simulink model "test"  (R2020b)
settings: Solver=FixedStepAuto  StartTime=0.0  StopTime=2000  RelTol=1e-3  EnableMultiTasking=on
undefined symbols (not defined in the file or in its folder): DiscIntNeverNeededParam
libraries: bbblueCommlib x15, simulink x7, bbblueBasicLib x4, bbblueSensorLib x1
settings Model: SimulationMode=external  ExtModeArchiveFileName=asd  ExtModeArchiveDirName=C:\Users\Zein\Desktop\gui  ExtModeIncDirWhenArm=on  Creator=Zein  LastModifiedBy=Zein
settings SolverCC: PositivePriorityOrder=on
settings OptimizationCC: EnhancedBackFolding=on  PassReuseOutputArgsAs=Individual arguments  ZeroExternalMemoryAtStartup=off  ZeroInternalMemoryAtStartup=off  MaxStackSize=64  OptimizeBlockOrder=speed  DifferentSizesBufferReuse=on  OptimizationCustomize=off  EfficientTunableParamExpr=on
settings DebuggingCC: ParameterTunabilityLossMsg=error
settings HardwareCC: ProdBitPerPointer=32  ProdBitPerSizeT=32  ProdBitPerPtrDiffT=32  ProdLargestAtomicInteger=Long  ProdLargestAtomicFloat=Double  ProdWordSize=32  ProdHWDeviceType=ARM Compatible->ARM Cortex
settings SFSimCC: MATLABDynamicMemAlloc=off
settings RTWCC: Description=Embedded Coder  SystemTargetFile=ert.tlc  HardwareBoard=BeagleBone Blue  TLCOptions="-aInlineSetEventsForThisBaseRateFcn=TLC_FALSE -aSuppressMultiTaskScheduler=TLC_FALSE  -aRateBasedStepFcn=0"  TemplateMakefile=ert_default_tmf  Toolchain=GNU GCC BeagleBone Blue
settings CodeAppCC: ForceParamTrailComments=on  IgnoreCustomStorageClasses=off  OperatorAnnotations=on  SimulinkDataObjDesc=on  SFDataObjDesc=on  InsertBlockDesc=on
settings ERTTargetCC: MatFileLogging=on  SupportVariableSizeSignals=on

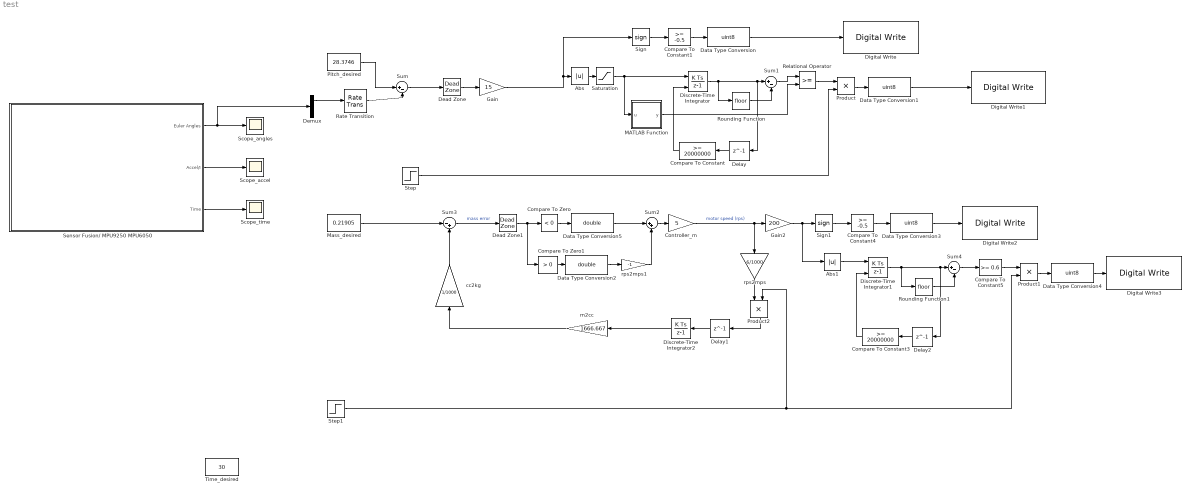
== system test ==
  Abs : Abs
  Abs1 : Abs
  Compare To Constant : simulink/Logic and Bit Operations/Compare To Constant  relop=>=  const=20000000  OutDataTypeStr=boolean
  Compare To Constant1 : simulink/Logic and Bit Operations/Compare To Constant  relop=>=  const=-0.5  OutDataTypeStr=boolean
  Compare To Constant3 : simulink/Logic and Bit Operations/Compare To Constant  relop=>=  const=20000000  OutDataTypeStr=boolean
  Compare To Constant4 : simulink/Logic and Bit Operations/Compare To Constant  relop=>=  const=-0.5  OutDataTypeStr=boolean
  Compare To Constant5 : simulink/Logic and Bit Operations/Compare To Constant  relop=>=  const=0.6  OutDataTypeStr=uint8
  Compare To Zero : simulink/Logic and Bit Operations/Compare To Zero  relop=<  OutDataTypeStr=boolean
  Compare To Zero1 : simulink/Logic and Bit Operations/Compare To Zero  relop=>  OutDataTypeStr=boolean
  Controller_m : Gain  Gain=5
  Data Type Conversion{,1,3..4} (4 alike) : DataTypeConversion  OutDataTypeStr=uint8
  Data Type Conversion2 : DataTypeConversion  OutDataTypeStr=double
  Data Type Conversion5 : DataTypeConversion  OutDataTypeStr=double
  Dead Zone : DeadZone  LowerValue=-5  UpperValue=5  SaturateOnIntegerOverflow=on
  Dead Zone1 : DeadZone  LowerValue=-0.0001  UpperValue=0.0001  SaturateOnIntegerOverflow=on
  Delay : Delay  DelayLength=1
  Delay1 : Delay  DelayLength=1  SampleTime=1/5000
  Delay2 : Delay  DelayLength=1
  Demux : Demux  Outputs=3
  Digital Write : bbblueBasicLib/Digital Write  GPIOSelect=GPIO3_1  Pin=49  Direction=output
      settings: SourceProductBaseCode=SC_BEAGLEBONE_BLUE
  Digital Write1 : bbblueBasicLib/Digital Write  GPIOSelect=GPIO3_2  Pin=49  Direction=output
      settings: SourceProductBaseCode=SC_BEAGLEBONE_BLUE
  Digital Write2 : bbblueBasicLib/Digital Write  GPIOSelect=GPIO1_17  Pin=49  Direction=output
      settings: SourceProductBaseCode=SC_BEAGLEBONE_BLUE
  Digital Write3 : bbblueBasicLib/Digital Write  GPIOSelect=GPIO1_25  Pin=49  Direction=output
      settings: SourceProductBaseCode=SC_BEAGLEBONE_BLUE
  Discrete-Time Integrator : DiscreteIntegrator  ExternalReset=rising  SampleTime=1/5000  ICPrevOutput=DiscIntNeverNeededParam  ICPrevScaledInput=DiscIntNeverNeededParam
  Discrete-Time Integrator1 : DiscreteIntegrator  ExternalReset=rising  SampleTime=1/5000  ICPrevOutput=DiscIntNeverNeededParam  ICPrevScaledInput=DiscIntNeverNeededParam
  Discrete-Time Integrator2 : DiscreteIntegrator  SampleTime=1/5000  ICPrevOutput=DiscIntNeverNeededParam  ICPrevScaledInput=DiscIntNeverNeededParam
  Gain : Gain  Gain=15
  Gain2 : Gain  Gain=200
  MATLAB Function : MATLAB Function  TreatAsAtomicUnit=on
  Mass_desired : Constant  Value=0.21905
  Pitch_desired : Constant  Value=28.3746
  Product : Product
  Product1 : Product
  Product2 : Product
  Rate Transition : RateTransition
  Relational Operator : RelationalOperator  OutDataTypeStr=boolean  RndMeth=Round
  Rounding Function : Rounding
  Rounding Function1 : Rounding
  Saturation : Saturate  UpperLimit=1000  LowerLimit=0
  Scope_accel : Scope
  Scope_angles : Scope
  Scope_time : Scope
  Sensor Fusion/ MPU9250 MPU6050 : Subsystem
  Sign : Signum
  Sign1 : Signum
  Step : Step  Time=31
  Step1 : Step  Time=3
  Sum : Sum  Inputs=|+-
  Sum1 : Sum  Inputs=|+-
  Sum2 : Sum  Inputs=|++
  Sum3 : Sum  Inputs=|-+
  Sum4 : Sum  Inputs=|+-
  Time_desired : Constant  Value=30
  cc2kg : Gain  Gain=1/1000
  m2cc : Gain  Gain=1666.667
  rps2mps : Gain  Gain=6/1000
  rps2mps1 : Gain  Gain=-1
  wires:
  Sensor Fusion/ MPU9250 MPU6050/1(Euler Angles) -> Scope_angles/1, Demux/1
  Sensor Fusion/ MPU9250 MPU6050/2(Accel/I) -> Scope_accel/1
  Sensor Fusion/ MPU9250 MPU6050/3(Time) -> Scope_time/1
  Pitch_desired/1 -> Sum/1
  Demux/1 -> Rate Transition/1
  Sum/1 -> Dead Zone/1
  Dead Zone/1 -> Gain/1
  Rate Transition/1 -> Sum/2
  Mass_desired/1 -> Sum3/1
  Saturation/1 -> MATLAB Function/1(u), Discrete-Time Integrator/1
  Sum1/1 -> Relational Operator/1
  MATLAB Function/1(y) -> Relational Operator/2
  Gain/1 -> Sign/1, Abs/1
  Abs/1 -> Saturation/1
  Step/1 -> Product/2
  Compare To Constant1/1 -> Data Type Conversion/1
  Discrete-Time Integrator/1 -> Delay/1, Sum1/1, Rounding Function/1
  Product/1 -> Data Type Conversion1/1
  Data Type Conversion/1 -> Digital Write/1
  Delay/1 -> Compare To Constant/1
  Compare To Constant/1 -> Discrete-Time Integrator/2
  Sign/1 -> Compare To Constant1/1
  Rounding Function/1 -> Sum1/2
  Data Type Conversion1/1 -> Digital Write1/1
  Relational Operator/1 -> Product/1
  Delay1/1 -> Discrete-Time Integrator2/1
  Dead Zone1/1 -> Compare To Zero1/1, Compare To Zero/1
  cc2kg/1 -> Sum3/2
  rps2mps/1 -> Product2/1
  rps2mps1/1 -> Sum2/2
  Compare To Constant5/1 -> Product1/1
  Sum2/1 -> Controller_m/1
  Controller_m/1 -> rps2mps/1, Gain2/1  "motor speed (rps)"
  Rounding Function1/1 -> Sum4/2
  Sign1/1 -> Compare To Constant4/1
  Product1/1 -> Data Type Conversion4/1
  Compare To Constant4/1 -> Data Type Conversion3/1
  Compare To Zero/1 -> Data Type Conversion5/1
  Data Type Conversion2/1 -> rps2mps1/1
  Sum3/1 -> Dead Zone1/1  "mass error"
  Discrete-Time Integrator2/1 -> m2cc/1
  Compare To Zero1/1 -> Data Type Conversion2/1
  Data Type Conversion5/1 -> Sum2/1
  Abs1/1 -> Discrete-Time Integrator1/1
  m2cc/1 -> cc2kg/1
  Sum4/1 -> Compare To Constant5/1
  Compare To Constant3/1 -> Discrete-Time Integrator1/2
  Discrete-Time Integrator1/1 -> Delay2/1, Sum4/1, Rounding Function1/1
  Delay2/1 -> Compare To Constant3/1
  Product2/1 -> Delay1/1
  Step1/1 -> Product2/2, Product1/2
  Gain2/1 -> Abs1/1, Sign1/1
  Data Type Conversion3/1 -> Digital Write2/1
  Data Type Conversion4/1 -> Digital Write3/1

== system test/Sensor Fusion// MPU9250 MPU6050 ==
  Digital Clock : DigitalClock  SampleTime=0.1
  If : If  IfExpression=u1 < 31
  Intialization : Subsystem  TreatAsAtomicUnit=on
  Running : Subsystem  TreatAsAtomicUnit=on
  Subsystem : Subsystem
  Subsystem1 : Subsystem
  Euler Angles : Outport
  Accel/I : Outport  Port=2
  Time : Outport  Port=3
  wires:
  Subsystem1/1(MPU9250 Data) -> Intialization/3(MPU9250 Data), Running/4(MPU9250 Data)  "MPU9250 Data"
  Intialization/1(MPU6050 Bias) -> Running/1(MPU6050 Biases)
  Subsystem/1(MPU6050 Data) -> Intialization/2(MPU6050 Data), Running/3(MPU6050 Data)  "MPU6050 Data"
  If/1 -> Intialization/Action
  If/2 -> Running/Action
  Running/1(Euler Angles) -> Euler Angles/1
  Intialization/2(MPU9250 Bias) -> Running/2(MPU9250 Biases)
  Running/2(Accel/I) -> Accel/I/1
  Digital Clock/1 -> Time/1, Intialization/1(Time), If/1

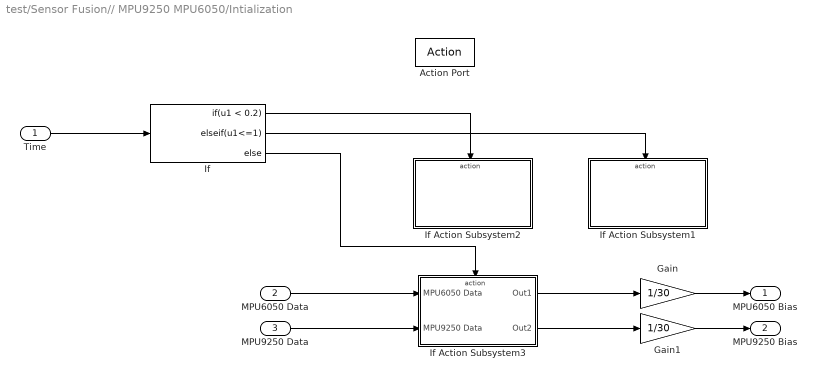
== system test/Sensor Fusion// MPU9250 MPU6050/Intialization ==
  Time : Inport
  MPU6050 Data : Inport  Port=2
  MPU9250 Data : Inport  Port=3
  Action Port : ActionPort  ActionPortLabel=if(u1 < 31)
  Gain : Gain  Gain=1/30
  Gain1 : Gain  Gain=1/30
  If : If  IfExpression=u1 < 0.2  ElseIfExpressions=u1<=1
  If Action Subsystem1 : Subsystem  TreatAsAtomicUnit=on
  If Action Subsystem2 : Subsystem  TreatAsAtomicUnit=on
  If Action Subsystem3 : Subsystem  TreatAsAtomicUnit=on
  MPU6050 Bias : Outport
  MPU9250 Bias : Outport  Port=2
  wires:
  Time/1 -> If/1
  If/1 -> If Action Subsystem2/Action
  If/2 -> If Action Subsystem1/Action
  If/3 -> If Action Subsystem3/Action
  If Action Subsystem3/1(Out1) -> Gain/1
  Gain/1 -> MPU6050 Bias/1
  If Action Subsystem3/2(Out2) -> Gain1/1
  Gain1/1 -> MPU9250 Bias/1
  MPU9250 Data/1 -> If Action Subsystem3/2(MPU9250 Data)
  MPU6050 Data/1 -> If Action Subsystem3/1(MPU6050 Data)

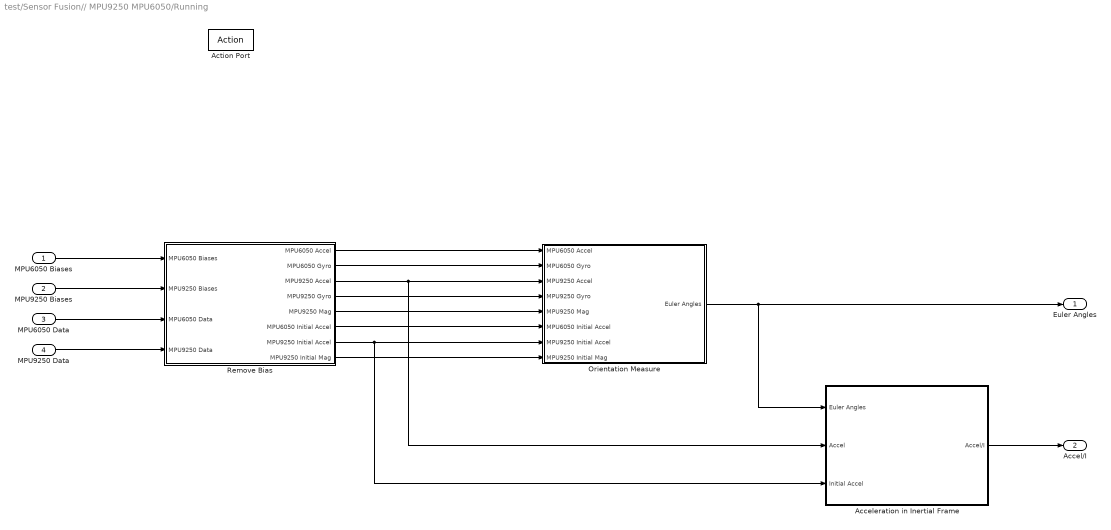
== system test/Sensor Fusion// MPU9250 MPU6050/Running ==
  MPU6050 Biases : Inport
  MPU9250 Biases : Inport  Port=2
  MPU6050 Data : Inport  Port=3
  MPU9250 Data : Inport  Port=4
  Action Port : ActionPort  ActionPortLabel=else
  Acceleration in Inertial Frame : Subsystem
  Orientation Measure : Subsystem
  Remove Bias : Subsystem
  Euler Angles : Outport
  Accel/I : Outport  Port=2
  wires:
  MPU6050 Biases/1 -> Remove Bias/1(MPU6050 Biases)
  MPU9250 Biases/1 -> Remove Bias/2(MPU9250 Biases)
  MPU9250 Data/1 -> Remove Bias/4(MPU9250 Data)
  MPU6050 Data/1 -> Remove Bias/3(MPU6050 Data)
  Remove Bias/1(MPU6050 Accel) -> Orientation Measure/1(MPU6050 Accel)
  Remove Bias/2(MPU6050 Gyro) -> Orientation Measure/2(MPU6050 Gyro)
  Remove Bias/3(MPU9250 Accel) -> Acceleration in Inertial Frame/2(Accel), Orientation Measure/3(MPU9250 Accel)
  Remove Bias/4(MPU9250 Gyro) -> Orientation Measure/4(MPU9250 Gyro)
  Remove Bias/5(MPU9250 Mag) -> Orientation Measure/5(" MPU9250 Mag")
  Remove Bias/6(MPU6050 Initial Accel) -> Orientation Measure/6(MPU6050 Initial Accel)
  Remove Bias/7(MPU9250 Initial Accel) -> Acceleration in Inertial Frame/3(Initial Accel), Orientation Measure/7(MPU9250 Initial Accel)
  Remove Bias/8(MPU9250 Initial Mag) -> Orientation Measure/8(MPU9250 Initial Mag)
  Orientation Measure/1(Euler Angles) -> Euler Angles/1, Acceleration in Inertial Frame/1(Euler Angles)
  Acceleration in Inertial Frame/1(Accel/I) -> Accel/I/1

== system test/Sensor Fusion// MPU9250 MPU6050/Subsystem ==
  MPU6050_Accelerometer : Subsystem
  MPU6050_Gyroscope : Subsystem
  Mux : Mux  Inputs=3
  Mux1 : Mux  Inputs=3
  Mux2 : Mux  Inputs=2
  MPU6050 Data : Outport
  wires:
  Mux/1 -> Mux2/1
  Mux1/1 -> Mux2/2
  MPU6050_Accelerometer/1(Out4) -> Mux/3  "x"
  MPU6050_Accelerometer/2(Out5) -> Mux/1  "y"
  MPU6050_Accelerometer/3(Out6) -> Mux/2  "z"
  MPU6050_Gyroscope/2(Out2) -> Mux1/1  "y"
  MPU6050_Gyroscope/1(Out1) -> Mux1/3  "x"
  MPU6050_Gyroscope/3(Out3) -> Mux1/2  "z"
  Mux2/1 -> MPU6050 Data/1

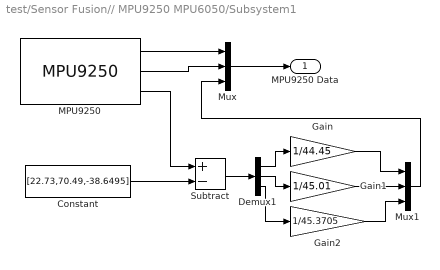
== system test/Sensor Fusion// MPU9250 MPU6050/Subsystem1 ==
  Constant : Constant  Value=[22.73,70.49,-38.6495]
  Demux1 : Demux  Outputs=3
  Gain : Gain  Gain=1/44.45
  Gain1 : Gain  Gain=1/45.01
  Gain2 : Gain  Gain=1/45.3705
  MPU9250 : bbblueSensorLib/MPU9250  OperationMode=Random  Accel=on  AngularRate=on  Ak8963Field=on  EulerAngles=on  Quat=off  AccelRange=2G  Acceldlpf=3  GyroRange=250 dps  Gyrodlpf=3  DmpOdr=200 Hz  SampleTime=0.1
      settings: SourceProductBaseCode=SC_BEAGLEBONE_BLUE
  Mux : Mux  Inputs=3
  Mux1 : Mux  Inputs=3
  Subtract : Sum  Inputs=+-
  MPU9250 Data : Outport
  wires:
  MPU9250/1 -> Mux/1
  MPU9250/2 -> Mux/2
  Mux/1 -> MPU9250 Data/1
  Constant/1 -> Subtract/2
  Subtract/1 -> Demux1/1
  MPU9250/3 -> Subtract/1
  Demux1/1 -> Gain/1
  Demux1/2 -> Gain1/1
  Demux1/3 -> Gain2/1
  Gain/1 -> Mux1/1
  Gain1/1 -> Mux1/2
  Gain2/1 -> Mux1/3
  Mux1/1 -> Mux/3

== system test/Sensor Fusion// MPU9250 MPU6050/Intialization/If Action Subsystem1 ==
  Action Port : ActionPort  ActionPortLabel=elseif(u1<=1)
  Constant : Constant  Value=0
  Constant1 : Constant  Value=3
  I2C Master Write : bbblueCommlib/I2C Master Write  I2CModule=1  Mode=Master  SlaveAddress=0x69  SlaveByteOrder=BigEndian  Direction=Transmitter  RegisterAddressMode=on  RegisterAddress=107  SlaveDataType=uint8  DataLength=1  NoAck=off  RepeatedStart=off  OutputStatus=off
      settings: SourceProductBaseCode=SC_BEAGLEBONE_BLUE
  I2C Master Write1 : bbblueCommlib/I2C Master Write  I2CModule=1  Mode=Master  SlaveAddress=0x69  SlaveByteOrder=BigEndian  Direction=Transmitter  RegisterAddressMode=on  RegisterAddress=26  SlaveDataType=uint8  DataLength=1  NoAck=off  RepeatedStart=off  OutputStatus=off
      settings: SourceProductBaseCode=SC_BEAGLEBONE_BLUE
  wires:
  Constant/1 -> I2C Master Write/1
  Constant1/1 -> I2C Master Write1/1

== system test/Sensor Fusion// MPU9250 MPU6050/Intialization/If Action Subsystem2 ==
  Action Port : ActionPort  ActionPortLabel=if(u1 < 0.2)
  Constant : Constant  Value=80
  I2C Master Write : bbblueCommlib/I2C Master Write  I2CModule=1  Mode=Master  SlaveAddress=0x69  SlaveByteOrder=BigEndian  Direction=Transmitter  RegisterAddressMode=on  RegisterAddress=107  SlaveDataType=uint8  DataLength=1  NoAck=off  RepeatedStart=off  OutputStatus=off
      settings: SourceProductBaseCode=SC_BEAGLEBONE_BLUE
  wires:
  Constant/1 -> I2C Master Write/1

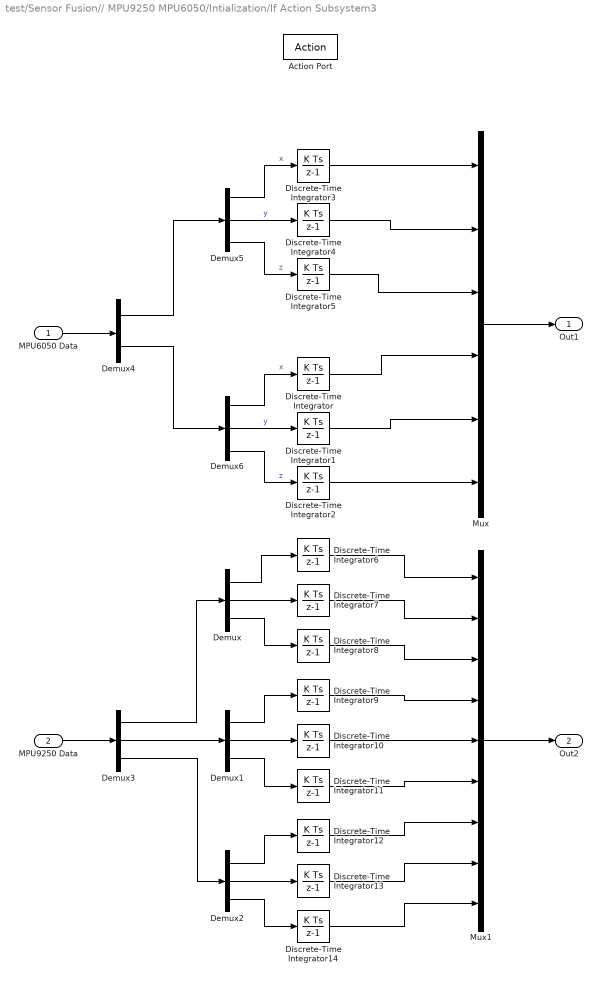
== system test/Sensor Fusion// MPU9250 MPU6050/Intialization/If Action Subsystem3 ==
  MPU6050 Data : Inport
  MPU9250 Data : Inport  Port=2
  Action Port : ActionPort  ActionPortLabel=else
  Demux{,1..3,5..6} (6 alike) : Demux  Outputs=3
  Demux4 : Demux  Outputs=2
  Discrete-Time Integrator{,1..14} (15 alike) : DiscreteIntegrator  SampleTime=-1  ICPrevOutput=DiscIntNeverNeededParam  ICPrevScaledInput=DiscIntNeverNeededParam
  Mux : Mux  Inputs=6
  Mux1 : Mux  Inputs=9
  Out1 : Outport
  Out2 : Outport  Port=2
  wires:
  Demux6/1 -> Discrete-Time Integrator/1  "x"
  Demux6/2 -> Discrete-Time Integrator1/1  "y"
  Demux6/3 -> Discrete-Time Integrator2/1  "z"
  Demux5/1 -> Discrete-Time Integrator3/1  "x"
  Demux5/2 -> Discrete-Time Integrator4/1  "y"
  Demux5/3 -> Discrete-Time Integrator5/1  "z"
  Mux/1 -> Out1/1
  Discrete-Time Integrator3/1 -> Mux/1
  Discrete-Time Integrator4/1 -> Mux/2
  Discrete-Time Integrator5/1 -> Mux/3
  Discrete-Time Integrator/1 -> Mux/4
  Discrete-Time Integrator1/1 -> Mux/5
  Discrete-Time Integrator2/1 -> Mux/6
  Demux3/1 -> Demux/1
  Demux3/2 -> Demux1/1
  Demux3/3 -> Demux2/1
  Mux1/1 -> Out2/1
  Demux/1 -> Discrete-Time Integrator6/1
  Demux/2 -> Discrete-Time Integrator7/1
  Demux/3 -> Discrete-Time Integrator8/1
  Demux1/1 -> Discrete-Time Integrator9/1
  Demux1/2 -> Discrete-Time Integrator10/1
  Demux1/3 -> Discrete-Time Integrator11/1
  Demux2/2 -> Discrete-Time Integrator13/1
  Demux2/1 -> Discrete-Time Integrator12/1
  Demux2/3 -> Discrete-Time Integrator14/1
  Discrete-Time Integrator10/1 -> Mux1/5
  Discrete-Time Integrator9/1 -> Mux1/4
  Discrete-Time Integrator8/1 -> Mux1/3
  Discrete-Time Integrator7/1 -> Mux1/2
  Discrete-Time Integrator6/1 -> Mux1/1
  Discrete-Time Integrator11/1 -> Mux1/6
  Discrete-Time Integrator12/1 -> Mux1/7
  Discrete-Time Integrator13/1 -> Mux1/8
  Discrete-Time Integrator14/1 -> Mux1/9
  MPU9250 Data/1 -> Demux3/1
  Demux4/1 -> Demux5/1
  Demux4/2 -> Demux6/1
  MPU6050 Data/1 -> Demux4/1

== system test/Sensor Fusion// MPU9250 MPU6050/Running/Acceleration in Inertial Frame ==
  Euler Angles : Inport
  Accel : Inport  Port=2
  Initial Accel : Inport  Port=3
  Gravity Measure B frame : Subsystem
  Gravity Measure_I frame : Subsystem
  Sum1 : Sum  Inputs=|+-
  Accel/I : Outport
  wires:
  Gravity Measure B frame/1(y) -> Sum1/2
  Initial Accel/1 -> Gravity Measure B frame/2(MPU9250 Initial Accel)
  Euler Angles/1 -> Gravity Measure_I frame/2(In2), Gravity Measure B frame/1(u)
  Sum1/1 -> Gravity Measure_I frame/1(u)
  Accel/1 -> Sum1/1
  Gravity Measure_I frame/1(y) -> Accel/I/1

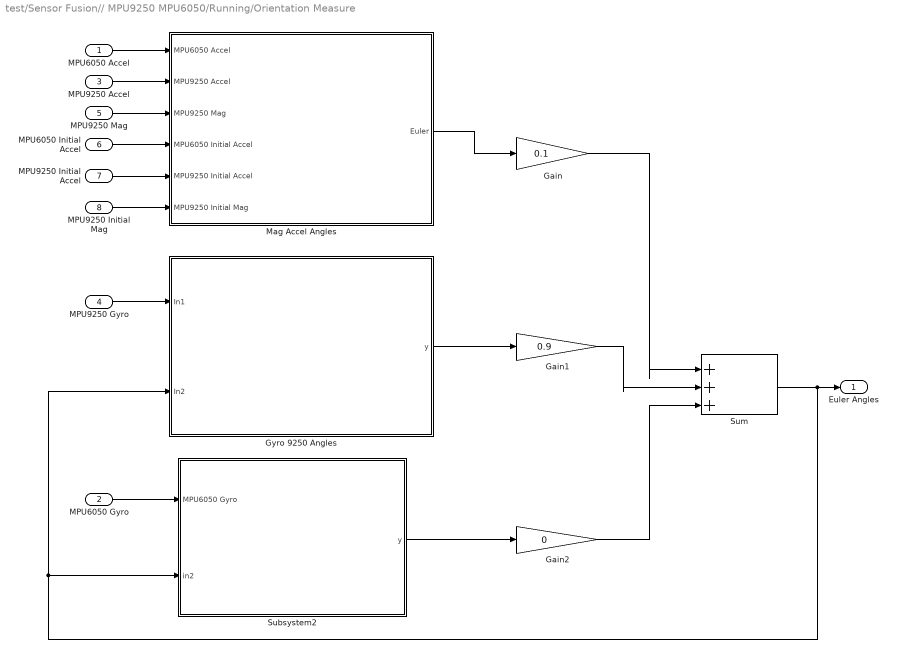
== system test/Sensor Fusion// MPU9250 MPU6050/Running/Orientation Measure ==
  MPU6050 Accel : Inport
  MPU6050 Gyro : Inport  Port=2
  MPU9250 Accel : Inport  Port=3
  MPU9250 Gyro : Inport  Port=4
  " MPU9250 Mag" : Inport  Port=5
  MPU6050 Initial Accel : Inport  Port=6
  MPU9250 Initial Accel : Inport  Port=7
  MPU9250 Initial Mag : Inport  Port=8
  Gain : Gain  Gain=0.1
  Gain1 : Gain  Gain=0.9
  Gain2 : Gain  Gain=0
  Gyro 9250 Angles : Subsystem
  Mag Accel Angles : Subsystem
  Subsystem2 : Subsystem
  Sum : Sum  Inputs=|+++
  Euler Angles : Outport
  wires:
  Gain2/1 -> Sum/3
  Mag Accel Angles/1(Euler) -> Gain/1
  Gain1/1 -> Sum/2
  Sum/1 -> Subsystem2/2(in2), Gyro 9250 Angles/2(In2), Euler Angles/1
  MPU9250 Gyro/1 -> Gyro 9250 Angles/1(In1)
  Gain/1 -> Sum/1
  MPU6050 Gyro/1 -> Subsystem2/1(MPU6050 Gyro)
  Gyro 9250 Angles/1(y) -> Gain1/1
  Subsystem2/1(y) -> Gain2/1
  MPU9250 Initial Accel/1 -> Mag Accel Angles/5(MPU9250 Initial Accel)
  MPU6050 Accel/1 -> Mag Accel Angles/1(MPU6050 Accel)
  MPU6050 Initial Accel/1 -> Mag Accel Angles/4(MPU6050 Initial Accel)
  MPU9250 Accel/1 -> Mag Accel Angles/2(MPU9250 Accel)
  " MPU9250 Mag"/1 -> Mag Accel Angles/3(" MPU9250 Mag")
  MPU9250 Initial Mag/1 -> Mag Accel Angles/6(MPU9250 Initial Mag)

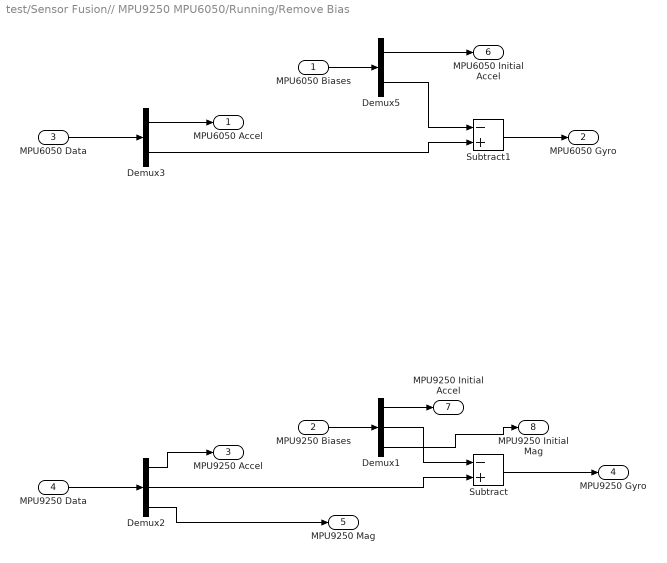
== system test/Sensor Fusion// MPU9250 MPU6050/Running/Remove Bias ==
  MPU6050 Biases : Inport
  MPU9250 Biases : Inport  Port=2
  MPU6050 Data : Inport  Port=3
  MPU9250 Data : Inport  Port=4
  Demux1 : Demux  Outputs=3
  Demux2 : Demux  Outputs=3
  Demux3 : Demux  Outputs=2
  Demux5 : Demux  Outputs=2
  Subtract : Sum  Inputs=-+
  Subtract1 : Sum  Inputs=-+
  MPU6050 Accel : Outport
  MPU6050 Gyro : Outport  Port=2
  MPU9250 Accel : Outport  Port=3
  MPU9250 Gyro : Outport  Port=4
  MPU9250 Mag : Outport  Port=5
  MPU6050 Initial Accel : Outport  Port=6
  MPU9250 Initial Accel : Outport  Port=7
  MPU9250 Initial Mag : Outport  Port=8
  wires:
  Demux5/2 -> Subtract1/1
  MPU9250 Data/1 -> Demux2/1
  Demux2/1 -> MPU9250 Accel/1
  MPU6050 Biases/1 -> Demux5/1
  Demux2/3 -> MPU9250 Mag/1
  Subtract1/1 -> MPU6050 Gyro/1
  MPU6050 Data/1 -> Demux3/1
  Demux3/2 -> Subtract1/2
  MPU9250 Biases/1 -> Demux1/1
  Demux3/1 -> MPU6050 Accel/1
  Demux1/2 -> Subtract/1
  Demux2/2 -> Subtract/2
  Subtract/1 -> MPU9250 Gyro/1
  Demux5/1 -> MPU6050 Initial Accel/1
  Demux1/1 -> MPU9250 Initial Accel/1
  Demux1/3 -> MPU9250 Initial Mag/1

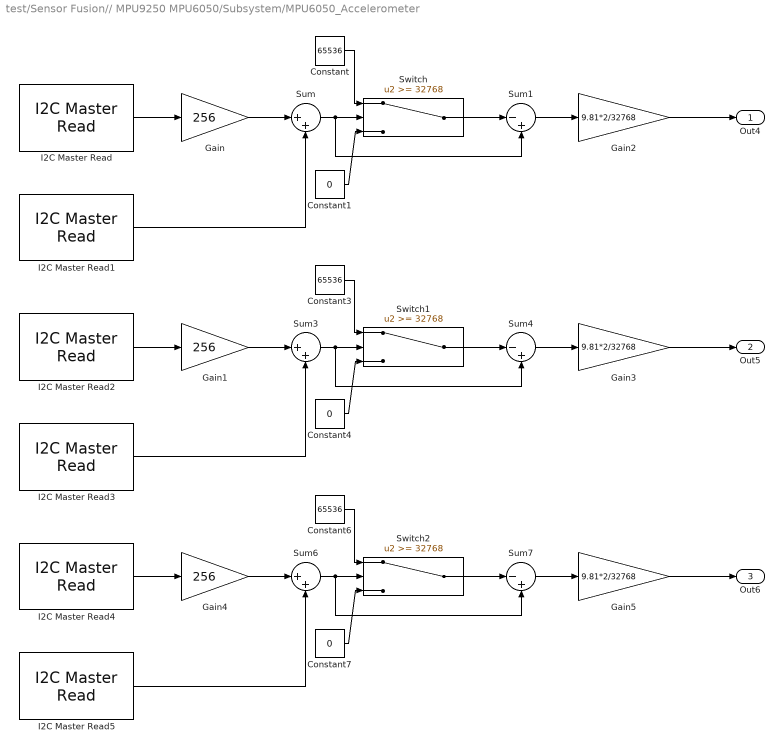
== system test/Sensor Fusion// MPU9250 MPU6050/Subsystem/MPU6050_Accelerometer ==
  Constant : Constant  Value=65536
  Constant1 : Constant  Value=0
  Constant3 : Constant  Value=65536
  Constant4 : Constant  Value=0
  Constant6 : Constant  Value=65536
  Constant7 : Constant  Value=0
  Gain : Gain  Gain=256
  Gain1 : Gain  Gain=256
  Gain2 : Gain  Gain=9.81*2/32768
  Gain3 : Gain  Gain=9.81*2/32768
  Gain4 : Gain  Gain=256
  Gain5 : Gain  Gain=9.81*2/32768
  I2C Master Read : bbblueCommlib/I2C Master Read  I2CModule=1  Mode=Master  SlaveAddress=0x69  SlaveByteOrder=BigEndian  Direction=Receiver  RegisterAddressMode=on  RegisterAddress=59  SlaveDataType=int8  DataLength=1  NoAck=off  RepeatedStart=off  OutputStatus=off  SampleTime=0.1
      settings: SourceProductBaseCode=SC_BEAGLEBONE_BLUE
  I2C Master Read1 : bbblueCommlib/I2C Master Read  I2CModule=1  Mode=Master  SlaveAddress=0x69  SlaveByteOrder=BigEndian  Direction=Receiver  RegisterAddressMode=on  RegisterAddress=60  SlaveDataType=int8  DataLength=1  NoAck=off  RepeatedStart=off  OutputStatus=off  SampleTime=0.1
      settings: SourceProductBaseCode=SC_BEAGLEBONE_BLUE
  I2C Master Read2 : bbblueCommlib/I2C Master Read  I2CModule=1  Mode=Master  SlaveAddress=0x69  SlaveByteOrder=BigEndian  Direction=Receiver  RegisterAddressMode=on  RegisterAddress=61  SlaveDataType=int8  DataLength=1  NoAck=off  RepeatedStart=off  OutputStatus=off  SampleTime=0.1
      settings: SourceProductBaseCode=SC_BEAGLEBONE_BLUE
  I2C Master Read3 : bbblueCommlib/I2C Master Read  I2CModule=1  Mode=Master  SlaveAddress=0x69  SlaveByteOrder=BigEndian  Direction=Receiver  RegisterAddressMode=on  RegisterAddress=62  SlaveDataType=int8  DataLength=1  NoAck=off  RepeatedStart=off  OutputStatus=off  SampleTime=0.1
      settings: SourceProductBaseCode=SC_BEAGLEBONE_BLUE
  I2C Master Read4 : bbblueCommlib/I2C Master Read  I2CModule=1  Mode=Master  SlaveAddress=0x69  SlaveByteOrder=BigEndian  Direction=Receiver  RegisterAddressMode=on  RegisterAddress=63  SlaveDataType=int8  DataLength=1  NoAck=off  RepeatedStart=off  OutputStatus=off  SampleTime=0.1
      settings: SourceProductBaseCode=SC_BEAGLEBONE_BLUE
  I2C Master Read5 : bbblueCommlib/I2C Master Read  I2CModule=1  Mode=Master  SlaveAddress=0x69  SlaveByteOrder=BigEndian  Direction=Receiver  RegisterAddressMode=on  RegisterAddress=64  SlaveDataType=int8  DataLength=1  NoAck=off  RepeatedStart=off  OutputStatus=off  SampleTime=0.1
      settings: SourceProductBaseCode=SC_BEAGLEBONE_BLUE
  Sum : Sum  Inputs=|++
  Sum1 : Sum  Inputs=|-+
  Sum3 : Sum  Inputs=|++
  Sum4 : Sum  Inputs=|-+
  Sum6 : Sum  Inputs=|++
  Sum7 : Sum  Inputs=|-+
  Switch : Switch  Threshold=32768
  Switch1 : Switch  Threshold=32768
  Switch2 : Switch  Threshold=32768
  Out4 : Outport
  Out5 : Outport  Port=2
  Out6 : Outport  Port=3
  wires:
  Constant/1 -> Switch/1
  I2C Master Read1/1 -> Sum/2
  I2C Master Read2/1 -> Gain1/1
  Sum/1 -> Switch/2, Sum1/2
  Sum4/1 -> Gain3/1
  Constant3/1 -> Switch1/1
  Sum6/1 -> Switch2/2, Sum7/2
  I2C Master Read4/1 -> Gain4/1
  Gain1/1 -> Sum3/1
  Switch/1 -> Sum1/1
  I2C Master Read5/1 -> Sum6/2
  Constant6/1 -> Switch2/1
  Switch2/1 -> Sum7/1
  Gain4/1 -> Sum6/1
  Switch1/1 -> Sum4/1
  I2C Master Read3/1 -> Sum3/2
  Gain2/1 -> Out4/1
  Constant1/1 -> Switch/3
  Constant4/1 -> Switch1/3
  Sum1/1 -> Gain2/1
  Sum7/1 -> Gain5/1
  Gain5/1 -> Out6/1
  I2C Master Read/1 -> Gain/1
  Gain/1 -> Sum/1
  Sum3/1 -> Sum4/2, Switch1/2
  Gain3/1 -> Out5/1
  Constant7/1 -> Switch2/3

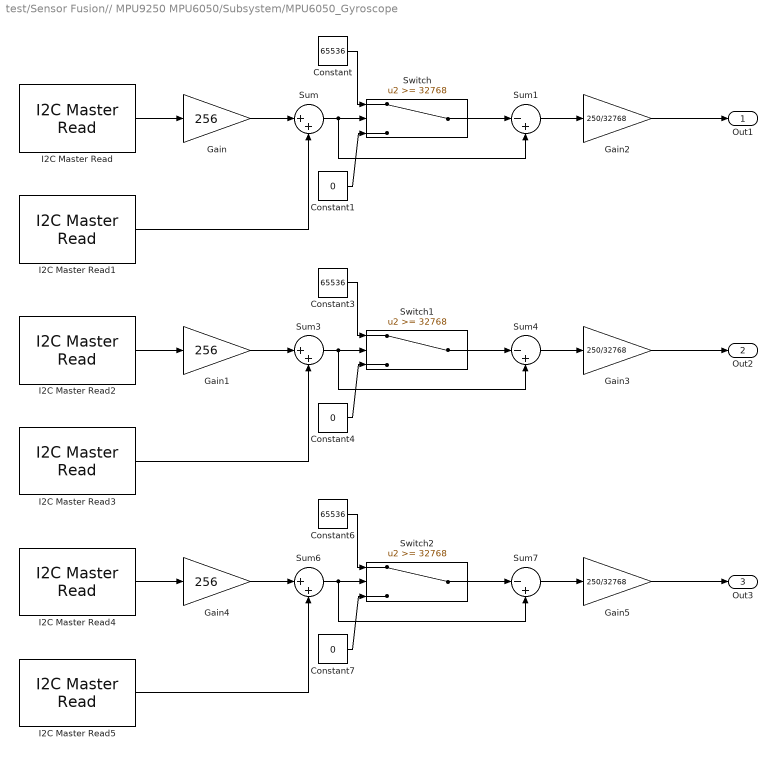
== system test/Sensor Fusion// MPU9250 MPU6050/Subsystem/MPU6050_Gyroscope ==
  Constant : Constant  Value=65536
  Constant1 : Constant  Value=0
  Constant3 : Constant  Value=65536
  Constant4 : Constant  Value=0
  Constant6 : Constant  Value=65536
  Constant7 : Constant  Value=0
  Gain : Gain  Gain=256
  Gain1 : Gain  Gain=256
  Gain2 : Gain  Gain=250/32768
  Gain3 : Gain  Gain=250/32768
  Gain4 : Gain  Gain=256
  Gain5 : Gain  Gain=250/32768
  I2C Master Read : bbblueCommlib/I2C Master Read  I2CModule=1  Mode=Master  SlaveAddress=0x69  SlaveByteOrder=BigEndian  Direction=Receiver  RegisterAddressMode=on  RegisterAddress=67  SlaveDataType=int8  DataLength=1  NoAck=off  RepeatedStart=off  OutputStatus=off  SampleTime=0.1
      settings: SourceProductBaseCode=SC_BEAGLEBONE_BLUE
  I2C Master Read1 : bbblueCommlib/I2C Master Read  I2CModule=1  Mode=Master  SlaveAddress=0x69  SlaveByteOrder=BigEndian  Direction=Receiver  RegisterAddressMode=on  RegisterAddress=68  SlaveDataType=int8  DataLength=1  NoAck=off  RepeatedStart=off  OutputStatus=off  SampleTime=0.1
      settings: SourceProductBaseCode=SC_BEAGLEBONE_BLUE
  I2C Master Read2 : bbblueCommlib/I2C Master Read  I2CModule=1  Mode=Master  SlaveAddress=0x69  SlaveByteOrder=BigEndian  Direction=Receiver  RegisterAddressMode=on  RegisterAddress=69  SlaveDataType=int8  DataLength=1  NoAck=off  RepeatedStart=off  OutputStatus=off  SampleTime=0.1
      settings: SourceProductBaseCode=SC_BEAGLEBONE_BLUE
  I2C Master Read3 : bbblueCommlib/I2C Master Read  I2CModule=1  Mode=Master  SlaveAddress=0x69  SlaveByteOrder=BigEndian  Direction=Receiver  RegisterAddressMode=on  RegisterAddress=70  SlaveDataType=int8  DataLength=1  NoAck=off  RepeatedStart=off  OutputStatus=off  SampleTime=0.1
      settings: SourceProductBaseCode=SC_BEAGLEBONE_BLUE
  I2C Master Read4 : bbblueCommlib/I2C Master Read  I2CModule=1  Mode=Master  SlaveAddress=0x69  SlaveByteOrder=BigEndian  Direction=Receiver  RegisterAddressMode=on  RegisterAddress=71  SlaveDataType=int8  DataLength=1  NoAck=off  RepeatedStart=off  OutputStatus=off  SampleTime=0.1
      settings: SourceProductBaseCode=SC_BEAGLEBONE_BLUE
  I2C Master Read5 : bbblueCommlib/I2C Master Read  I2CModule=1  Mode=Master  SlaveAddress=0x69  SlaveByteOrder=BigEndian  Direction=Receiver  RegisterAddressMode=on  RegisterAddress=72  SlaveDataType=int8  DataLength=1  NoAck=off  RepeatedStart=off  OutputStatus=off  SampleTime=0.1
      settings: SourceProductBaseCode=SC_BEAGLEBONE_BLUE
  Sum : Sum  Inputs=|++
  Sum1 : Sum  Inputs=|-+
  Sum3 : Sum  Inputs=|++
  Sum4 : Sum  Inputs=|-+
  Sum6 : Sum  Inputs=|++
  Sum7 : Sum  Inputs=|-+
  Switch : Switch  Threshold=32768
  Switch1 : Switch  Threshold=32768
  Switch2 : Switch  Threshold=32768
  Out1 : Outport
  Out2 : Outport  Port=2
  Out3 : Outport  Port=3
  wires:
  I2C Master Read3/1 -> Sum3/2
  Sum4/1 -> Gain3/1
  Sum/1 -> Switch/2, Sum1/2
  I2C Master Read/1 -> Gain/1
  Sum3/1 -> Sum4/2, Switch1/2
  I2C Master Read1/1 -> Sum/2
  Constant/1 -> Switch/1
  Gain/1 -> Sum/1
  Sum6/1 -> Switch2/2, Sum7/2
  Constant1/1 -> Switch/3
  Switch/1 -> Sum1/1
  Sum1/1 -> Gain2/1
  I2C Master Read4/1 -> Gain4/1
  Switch2/1 -> Sum7/1
  I2C Master Read2/1 -> Gain1/1
  Switch1/1 -> Sum4/1
  Constant4/1 -> Switch1/3
  Gain1/1 -> Sum3/1
  Constant3/1 -> Switch1/1
  Gain4/1 -> Sum6/1
  Sum7/1 -> Gain5/1
  Gain2/1 -> Out1/1
  Constant6/1 -> Switch2/1
  I2C Master Read5/1 -> Sum6/2
  Constant7/1 -> Switch2/3
  Gain3/1 -> Out2/1
  Gain5/1 -> Out3/1

== system test/Sensor Fusion// MPU9250 MPU6050/Running/Acceleration in Inertial Frame/Gravity Measure B frame ==
  u : Inport
  MPU9250 Initial Accel : Inport  Port=2
  MATLAB Function : MATLAB Function  TreatAsAtomicUnit=on
  Mux : Mux  Inputs=2
  y : Outport
  wires:
  u/1 -> Mux/1
  MATLAB Function/1(y) -> y/1
  MPU9250 Initial Accel/1 -> Mux/2
  Mux/1 -> MATLAB Function/1(u)

== system test/Sensor Fusion// MPU9250 MPU6050/Running/Acceleration in Inertial Frame/Gravity Measure_I frame ==
  u : Inport
  In2 : Inport  Port=2
  MATLAB Function : MATLAB Function  TreatAsAtomicUnit=on
  Mux : Mux  Inputs=2
  y : Outport
  wires:
  MATLAB Function/1(y) -> y/1
  u/1 -> Mux/1
  In2/1 -> Mux/2
  Mux/1 -> MATLAB Function/1(u)

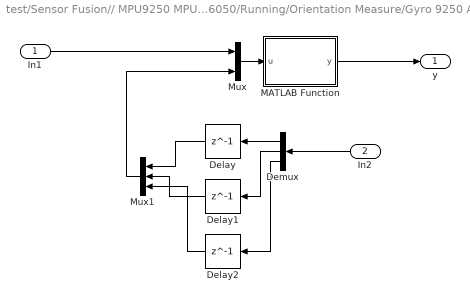
== system test/Sensor Fusion// MPU9250 MPU6050/Running/Orientation Measure/Gyro 9250 Angles ==
  In1 : Inport
  In2 : Inport  Port=2
  Delay : Delay  DelayLength=1
  Delay1 : Delay  DelayLength=1
  Delay2 : Delay  DelayLength=1
  Demux : Demux  Outputs=3
  MATLAB Function : MATLAB Function  TreatAsAtomicUnit=on
  Mux : Mux  Inputs=2
  Mux1 : Mux  Inputs=3
  y : Outport
  wires:
  Delay/1 -> Mux1/1
  In1/1 -> Mux/1
  Mux1/1 -> Mux/2
  Mux/1 -> MATLAB Function/1(u)
  Demux/2 -> Delay1/1
  Delay1/1 -> Mux1/2
  Demux/1 -> Delay/1
  Delay2/1 -> Mux1/3
  Demux/3 -> Delay2/1
  MATLAB Function/1(y) -> y/1
  In2/1 -> Demux/1

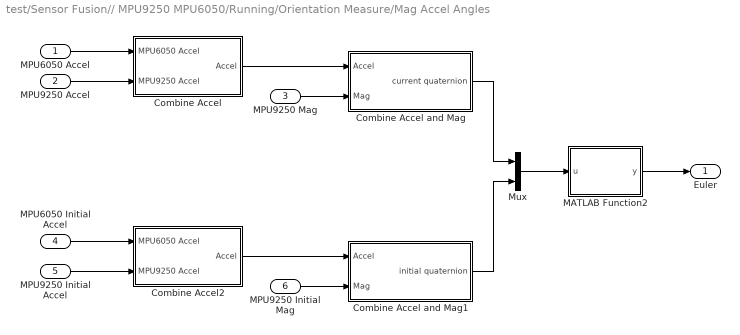
== system test/Sensor Fusion// MPU9250 MPU6050/Running/Orientation Measure/Mag Accel Angles ==
  MPU6050 Accel : Inport
  MPU9250 Accel : Inport  Port=2
  " MPU9250 Mag" : Inport  Port=3
  MPU6050 Initial Accel : Inport  Port=4
  MPU9250 Initial Accel : Inport  Port=5
  MPU9250 Initial Mag : Inport  Port=6
  Combine Accel : Subsystem
  Combine Accel and Mag : Subsystem
  Combine Accel and Mag1 : Subsystem
  Combine Accel2 : Subsystem
  MATLAB Function2 : MATLAB Function  TreatAsAtomicUnit=on
  Mux : Mux  Inputs=2
  Euler : Outport
  wires:
  " MPU9250 Mag"/1 -> Combine Accel and Mag/2(" Mag")
  Combine Accel/1(Accel) -> Combine Accel and Mag/1(Accel)
  Combine Accel and Mag1/1(initial quaternion) -> Mux/2
  MPU6050 Initial Accel/1 -> Combine Accel2/1(MPU6050 Accel)
  Mux/1 -> MATLAB Function2/1(u)
  MPU9250 Accel/1 -> Combine Accel/2(MPU9250 Accel)
  Combine Accel2/1(Accel) -> Combine Accel and Mag1/1(Accel)
  Combine Accel and Mag/1(current quaternion) -> Mux/1
  MPU6050 Accel/1 -> Combine Accel/1(MPU6050 Accel)
  MPU9250 Initial Accel/1 -> Combine Accel2/2(MPU9250 Accel)
  MPU9250 Initial Mag/1 -> Combine Accel and Mag1/2(" Mag")
  MATLAB Function2/1(y) -> Euler/1

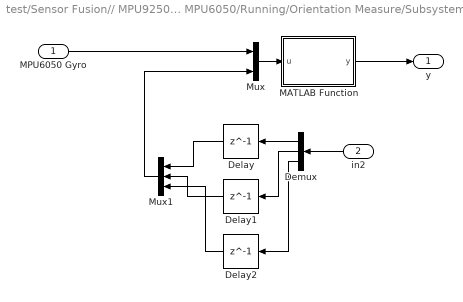
== system test/Sensor Fusion// MPU9250 MPU6050/Running/Orientation Measure/Subsystem2 ==
  MPU6050 Gyro : Inport
  in2 : Inport  Port=2
  Delay : Delay  DelayLength=1
  Delay1 : Delay  DelayLength=1
  Delay2 : Delay  DelayLength=1
  Demux : Demux  Outputs=3
  MATLAB Function : MATLAB Function  TreatAsAtomicUnit=on
  Mux : Mux  Inputs=2
  Mux1 : Mux  Inputs=3
  y : Outport
  wires:
  MATLAB Function/1(y) -> y/1
  Demux/3 -> Delay2/1
  Delay2/1 -> Mux1/3
  Demux/1 -> Delay/1
  Delay1/1 -> Mux1/2
  Demux/2 -> Delay1/1
  Mux/1 -> MATLAB Function/1(u)
  Mux1/1 -> Mux/2
  MPU6050 Gyro/1 -> Mux/1
  Delay/1 -> Mux1/1
  in2/1 -> Demux/1

== system test/Sensor Fusion// MPU9250 MPU6050/Running/Orientation Measure/Mag Accel Angles/Combine Accel ==
  MPU6050 Accel : Inport
  MPU9250 Accel : Inport  Port=2
  Add : Sum
  Gain : Gain  Gain=1/2
  Accel : Outport
  wires:
  MPU9250 Accel/1 -> Add/2
  Add/1 -> Gain/1
  Gain/1 -> Accel/1
  MPU6050 Accel/1 -> Add/1

== system test/Sensor Fusion// MPU9250 MPU6050/Running/Orientation Measure/Mag Accel Angles/Combine Accel and Mag ==
  Accel : Inport
  " Mag" : Inport  Port=2
  MATLAB Function : MATLAB Function  TreatAsAtomicUnit=on
  MATLAB Function1 : MATLAB Function  TreatAsAtomicUnit=on
  MATLAB Function2 : MATLAB Function  TreatAsAtomicUnit=on
  Mux : Mux  Inputs=2
  current quaternion : Outport
  wires:
  Accel/1 -> MATLAB Function/1(u)
  " Mag"/1 -> MATLAB Function1/1(u)
  Mux/1 -> MATLAB Function2/1(u)
  MATLAB Function2/1(y) -> current quaternion/1
  MATLAB Function/1(y) -> Mux/1
  MATLAB Function1/1(y) -> Mux/2

== system test/Sensor Fusion// MPU9250 MPU6050/Running/Orientation Measure/Mag Accel Angles/Combine Accel and Mag1 ==
  Accel : Inport
  " Mag" : Inport  Port=2
  MATLAB Function : MATLAB Function  TreatAsAtomicUnit=on
  MATLAB Function1 : MATLAB Function  TreatAsAtomicUnit=on
  MATLAB Function2 : MATLAB Function  TreatAsAtomicUnit=on
  Mux : Mux  Inputs=2
  initial quaternion : Outport
  wires:
  MATLAB Function1/1(y) -> Mux/2
  MATLAB Function/1(y) -> Mux/1
  MATLAB Function2/1(y) -> initial quaternion/1
  Mux/1 -> MATLAB Function2/1(u)
  " Mag"/1 -> MATLAB Function1/1(u)
  Accel/1 -> MATLAB Function/1(u)

== system test/Sensor Fusion// MPU9250 MPU6050/Running/Orientation Measure/Mag Accel Angles/Combine Accel2 ==
  MPU6050 Accel : Inport
  MPU9250 Accel : Inport  Port=2
  Add : Sum
  Gain : Gain  Gain=1/2
  Accel : Outport
  wires:
  Gain/1 -> Accel/1
  Add/1 -> Gain/1
  MPU9250 Accel/1 -> Add/2
  MPU6050 Accel/1 -> Add/1

== matlab function test/Sensor Fusion// MPU9250 MPU6050/Running/Orientation Measure/Mag Accel Angles/Combine Accel and Mag/MATLAB Function ==
  data: u input; y output
function y = fcn(u)

y=u/norm(u);

== matlab function test/Sensor Fusion// MPU9250 MPU6050/Running/Orientation Measure/Mag Accel Angles/Combine Accel and Mag/MATLAB Function2 ==
  data: u input; y output
function y = fcn(u)

accel=[u(1);u(2);u(3)];
mag=[u(5);u(4);-u(6)];
q = ecompass(accel',mag');
y=compact(q);


% 
% theta=asin(-R(3,1));
% psi=atan2(R(2,1),R(1,1));
% phi=atan2(R(3,2),R(3,3));
% euler=[phi;theta;psi];


% r = ecompass(accel',mag','rotmat')';
% theta = -asin(r(1,3));
% psi = atan2(r(2,3)/cos(theta),r(3,3)/cos(theta));
% rho = atan2(r(1,2)/cos(theta),r(1,1)/cos(theta));
% euler = rad2deg([rho,theta,psi]);

== matlab function test/Sensor Fusion// MPU9250 MPU6050/Running/Orientation Measure/Gyro 9250 Angles/MATLAB Function ==
  data: u input; y output
function y = fcn(u)

if(length(u)==6) 
    Gyro=[u(1);u(2);u(3)];
    Previous=[u(4);u(5);u(6)];

    ph=Previous(1);
    tet=Previous(2);

    R1=[1,sind(ph)*tand(tet),cosd(ph)*tand(tet);
        0,cosd(ph),-sind(ph);
        0,sind(ph)/cosd(tet),cosd(ph)/cosd(tet)];

    dt=0.1;

    New=Previous+R1*Gyro*dt;
else
    New=[0;0;0];
end

y = New;

== matlab function test/Sensor Fusion// MPU9250 MPU6050/Running/Orientation Measure/Subsystem2/MATLAB Function ==
  data: u input; y output
function y = fcn(u)

if(length(u)==6) 
    Gyro=[u(1);u(2);u(3)];
    Previous=[u(4);u(5);u(6)];

    ph=Previous(1);
    tet=Previous(2);

    R1=[1,sind(ph)*tand(tet),cosd(ph)*tand(tet);
        0,cosd(ph),-sind(ph);
        0,sind(ph)/cosd(tet),cosd(ph)/cosd(tet)];

    dt=0.1;

    New=Previous+R1*Gyro*dt;
else
    New=[0;0;0];
end

y = New;

== matlab function test/MATLAB Function ==
  data: u input; y output
function y = fcn(u)
    if u<260 
        a=0.95;
    elseif u<550
        a=0.7;
    elseif u<650
        a=0.6;
    else
        a=0.4;
    end
y = a;

== matlab function test/Sensor Fusion// MPU9250 MPU6050/Running/Orientation Measure/Mag Accel Angles/Combine Accel and Mag1/MATLAB Function ==
  data: u input; y output
function y = fcn(u)

y=u/norm(u);

== matlab function test/Sensor Fusion// MPU9250 MPU6050/Running/Orientation Measure/Mag Accel Angles/Combine Accel and Mag1/MATLAB Function1 ==
  data: u input; y output
function y = fcn(u)

y=u/norm(u);

== matlab function test/Sensor Fusion// MPU9250 MPU6050/Running/Orientation Measure/Mag Accel Angles/Combine Accel and Mag1/MATLAB Function2 ==
  data: u input; y output
function y = fcn(u)

accel=[u(1);u(2);u(3)];
mag=[u(5);u(4);-u(6)];
q = ecompass(accel',mag');

y=compact(q);

== matlab function test/Sensor Fusion// MPU9250 MPU6050/Running/Orientation Measure/Mag Accel Angles/Combine Accel and Mag/MATLAB Function1 ==
  data: u input; y output
function y = fcn(u)

y=u/norm(u);

== matlab function test/Sensor Fusion// MPU9250 MPU6050/Running/Orientation Measure/Mag Accel Angles/MATLAB Function2 ==
  data: u input; y output
function y = fcn(u)

q2=[u(1),u(2),u(3),u(4)];
q1=[u(5),u(6),u(7),u(8)];

Q1=quaternion(q1);
Q2=quaternion(q2);

R1 = rotmat(Q1,'frame');
R2 = rotmat(Q2,'frame');

R=R1*R2';

theta=asin(-R(3,1));
psi=atan2(R(2,1)/cos(theta),R(1,1)/cos(theta));
phi=atan2(R(3,2)/cos(theta),R(3,3)/cos(theta));
euler=[phi;theta;psi]*180/pi;

y=euler;


% 
% theta=asin(-R(3,1));
% psi=atan2(R(2,1),R(1,1));
% phi=atan2(R(3,2),R(3,3));
% euler=[phi;theta;psi];


% r = ecompass(accel',mag','rotmat')';
% theta = -asin(r(1,3));
% psi = atan2(r(2,3)/cos(theta),r(3,3)/cos(theta));
% rho = atan2(r(1,2)/cos(theta),r(1,1)/cos(theta));
% euler = rad2deg([rho,theta,psi]);

== matlab function test/Sensor Fusion// MPU9250 MPU6050/Running/Acceleration in Inertial Frame/Gravity Measure B frame/MATLAB Function ==
  data: u input; y output
function y = fcn(u)

if(length(u)==6)
    euler=[u(1);u(2);u(3)];
    q=quaternion(euler', 'eulerd','XYZ','point');
    r=rotmat(q,'point');
    g=[u(4);u(5);u(6)];

    g1=r'*g;
else
    g1=[0;0;0];
end


y = g1;

== matlab function test/Sensor Fusion// MPU9250 MPU6050/Running/Acceleration in Inertial Frame/Gravity Measure_I frame/MATLAB Function ==
  data: u input; y output
function y = fcn(u)

if(length(u)==6)
    g1=[u(1);u(2);u(3)];
    euler=[u(4);u(5);u(6)];
    q=quaternion(euler', 'eulerd','XYZ','point');
    r=rotmat(q,'point');
%     g=[0;0;10];
    g=r*g1;
else
    g=[0;0;0];
end


y = g;
